simulink library "Surface_Mu_Axle2_Constant"  (R2023b)
settings: Solver=VariableStepAuto  StartTime=0.0  StopTime=10.0  RelTol=1e-3
undefined symbols (not defined in the file or in its folder): Scene
libraries: Tire_Utilities x4
Description:
  | Simscape Vehicle Templates Library
  | 
  | Copyright 2018-2024 The MathWorks, Inc.
settings Model: Creator=smiller  LastModifiedBy=smiller
settings ModelReferenceCC: EnableRefExpFcnMdlSchedulingChecks=on

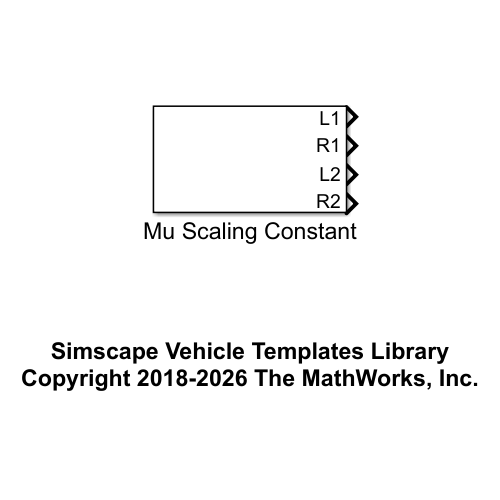
[thumbnail: Simulink's stored preview of the top-level diagram]
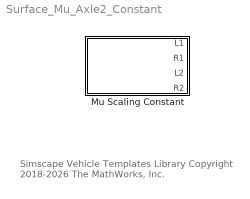
== system Surface_Mu_Axle2_Constant ==
  note: Simscape Vehicle Templates Library
      | Copyright 2018-2026 The MathWorks, Inc.
  Mu Scaling Constant : Subsystem  mask(Friction Scaling Coefficient Constant (Two Axle)){scaleCoefficient=Scene.Mu_Scaling.constant}
      mask prompts: scaleCoefficient "Friction Scaling Coefficient (0-1)"
      mask help: Friction scaling coefficient factor set to constant.

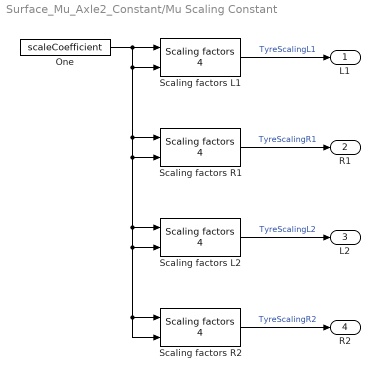
== system Surface_Mu_Axle2_Constant/Mu Scaling Constant ==
  One : Constant  Value=scaleCoefficient  OutDataTypeStr=Inherit: Inherit via back propagation
  Scaling factors L1 : Tire_Utilities/Scaling factors 4  LKX=1  LKY=1  LKYC=1  LTR=1  LKZC=1
  Scaling factors L2 : Tire_Utilities/Scaling factors 4  LKX=1  LKY=1  LKYC=1  LTR=1  LKZC=1
  Scaling factors R1 : Tire_Utilities/Scaling factors 4  LKX=1  LKY=1  LKYC=1  LTR=1  LKZC=1
  Scaling factors R2 : Tire_Utilities/Scaling factors 4  LKX=1  LKY=1  LKYC=1  LTR=1  LKZC=1
  L1 : Outport  VectorParamsAs1DForOutWhenUnconnected=off
  R1 : Outport  Port=2  VectorParamsAs1DForOutWhenUnconnected=off
  L2 : Outport  Port=3  VectorParamsAs1DForOutWhenUnconnected=off
  R2 : Outport  Port=4  VectorParamsAs1DForOutWhenUnconnected=off
  wires:
  Scaling factors L2/1 -> L2/1  "TyreScalingL2"
  Scaling factors R2/1 -> R2/1  "TyreScalingR2"
  Scaling factors R1/1 -> R1/1  "TyreScalingR1"
  One/1 -> Scaling factors R2/2, Scaling factors R2/1, Scaling factors L2/2, Scaling factors L2/1, Scaling factors R1/2, Scaling factors R1/1, Scaling factors L1/2, Scaling factors L1/1
  Scaling factors L1/1 -> L1/1  "TyreScalingL1"
